simulink model "my_qpsk_simulink"  (R2022a)
settings: Solver=ode45  StartTime=0.0  StopTime=10.0  RelTol=1e-3  EnableMultiTasking=on
PreLoadFcn:
  | clc;
  | clear;
  | fs = 56e06;
  | f_clk = fs*6;
  | 
  | f_0 = 70e06;
  | f_c = f_0 - fs;
  | f_dds_out = f_c;
libraries: dsparch4 x4, dspxfrm3 x2, commchan3 x1, commsynccomp2 x1, commrandsrc2 x1, simulink x1, commdigbbndpm3 x1, dspsrcs4 x1
settings Model: Creator=laohe  LastModifiedBy=imlao
settings SolverCC: AlgebraicLoopSolver=TrustRegion
settings DataIOCC: LimitDataPoints=on  SaveFormat=Array  SignalLoggingSaveFormat=ModelDataLogs  ReturnWorkspaceOutputs=off
settings OptimizationCC: ExpressionDepthLimit=2147483647  LifeSpan=inf
settings DebuggingCC: UnderspecifiedInitializationDetection=Classic  MergeDetectMultiDrivingBlocksExec=none  SolverPrmCheckMsg=warning  FcnCallInpInsideContextMsg=warning  UnconnectedInputMsg=warning  UnconnectedOutputMsg=warning  UnconnectedLineMsg=warning  StateNameClashWarn=warning  SFUnexpectedBacktrackingDiag=warning  SFNoUnconditionalDefaultTransitionDiag=warning  SFExecutionAtInitializationDiag=none  SFMachineParentedDataDiag=warning  ArithmeticOperatorsInVariantConditions=warning
settings HardwareCC: ProdBitPerPointer=32  ProdBitPerSizeT=32  ProdBitPerPtrDiffT=32  ProdLargestAtomicFloat=None  ProdIntDivRoundTo=Undefined  ProdEndianess=Unspecified  ProdWordSize=32  ProdHWDeviceType=32-bit Generic
settings ModelReferenceCC: PropagateSignalLabelsOutOfModel=off
settings SFSimCC: SimUseLocalCustomCode=off  CustomCodeUndefinedFunction=UseInterfaceOnly
settings RTWCC: RTWUseLocalCustomCode=off
settings CodeAppCC: StateflowObjectComments=on
settings GRTTargetCC: TargetLangStandard=C89/C90 (ANSI)
settings ConfigComp: CovMetricSettings=dw  CovSaveCumulativeToWorkspaceVar=on  CovSaveSingleToWorkspaceVar=on  CovExternalEMLEnable=off

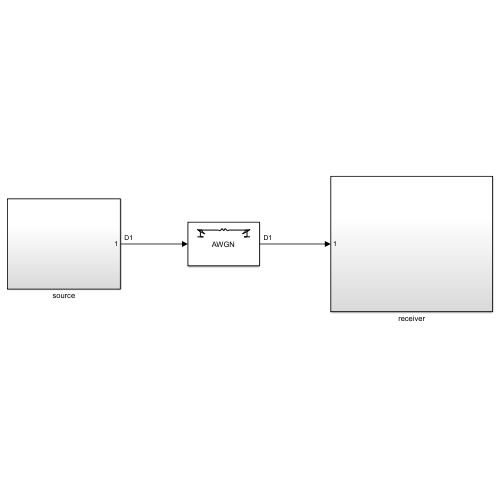
[thumbnail: Simulink's stored preview of the top-level diagram]
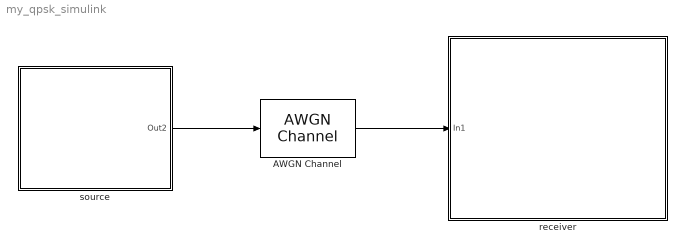
== system my_qpsk_simulink ==
  AWGN Channel : commchan3/AWGN Channel  InputProcessing=Columns as channels (frame based)  seed=67  noiseMode="Signal to noise ratio  (SNR)"  EbNodB=10  EsNodB=10  SNRdB=111  bitsPerSym=2  Ps=1  Tsym=1/2e06  variance=1
  receiver : Subsystem
  source : Subsystem
  wires:
  source/1(Out2) -> AWGN Channel/1
  AWGN Channel/1 -> receiver/1(In1)

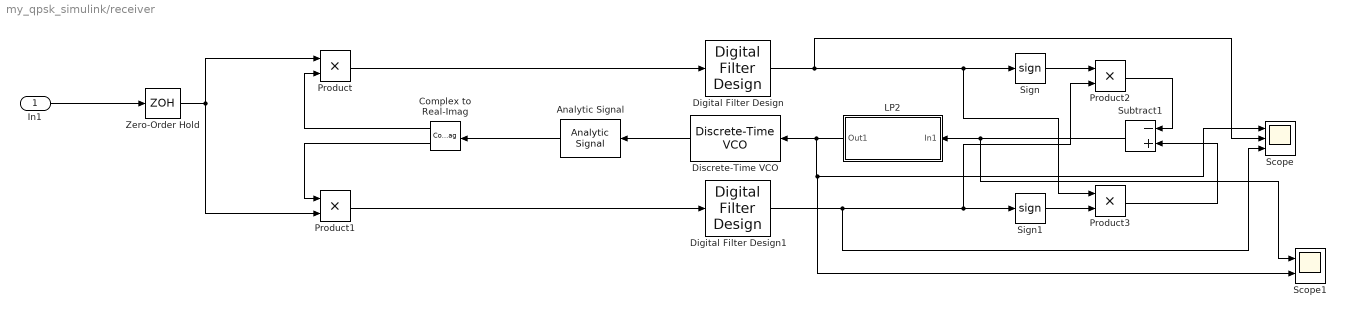
== system my_qpsk_simulink/receiver ==
  In1 : Inport
  Analytic Signal : dspxfrm3/Analytic Signal  N=100  InputProcessing=Columns as channels (frame based)
      settings: SourceProductBaseCode=DS
  Complex to Real-Imag : ComplexToRealImag
  Digital Filter Design : dsparch4/Digital Filter Design  mwdsp_browser_bugfix_var=off
  Digital Filter Design1 : dsparch4/Digital Filter Design  mwdsp_browser_bugfix_var=off
  Discrete-Time VCO : commsynccomp2/Discrete-Time VCO  Ac=1  Fc=f_dds_out  Kc=10000  Ph=0  ts=1/fs
      settings: SourceProductBaseCode=CM
  LP2 : Subsystem
  Product{,1..3} (4 alike) : Product  RndMeth=Zero
  Scope : Scope  NumInputPorts=3
  Scope1 : Scope  NumInputPorts=2
  Sign : Signum
  Sign1 : Signum
  Subtract1 : Sum  Inputs=-+
  Zero-Order Hold : ZeroOrderHold  SampleTime=1/fs
  wires:
  Analytic Signal/1 -> Complex to Real-Imag/1
  Complex to Real-Imag/1 -> Product/2
  Discrete-Time VCO/1 -> Analytic Signal/1
  Complex to Real-Imag/2 -> Product1/1
  In1/1 -> Zero-Order Hold/1
  Product1/1 -> Digital Filter Design1/1
  Product/1 -> Digital Filter Design/1
  Zero-Order Hold/1 -> Product1/2, Product/1
  Digital Filter Design/1 -> Scope/2, Product3/1, Sign/1
  LP2/1(Out1) -> Scope1/2, Scope/1, Discrete-Time VCO/1
  Sign/1 -> Product2/1
  Digital Filter Design1/1 -> Scope/3, Product2/2, Sign1/1
  Sign1/1 -> Product3/2
  Product2/1 -> Subtract1/1
  Product3/1 -> Subtract1/2
  Subtract1/1 -> Scope1/1, LP2/1(In1)

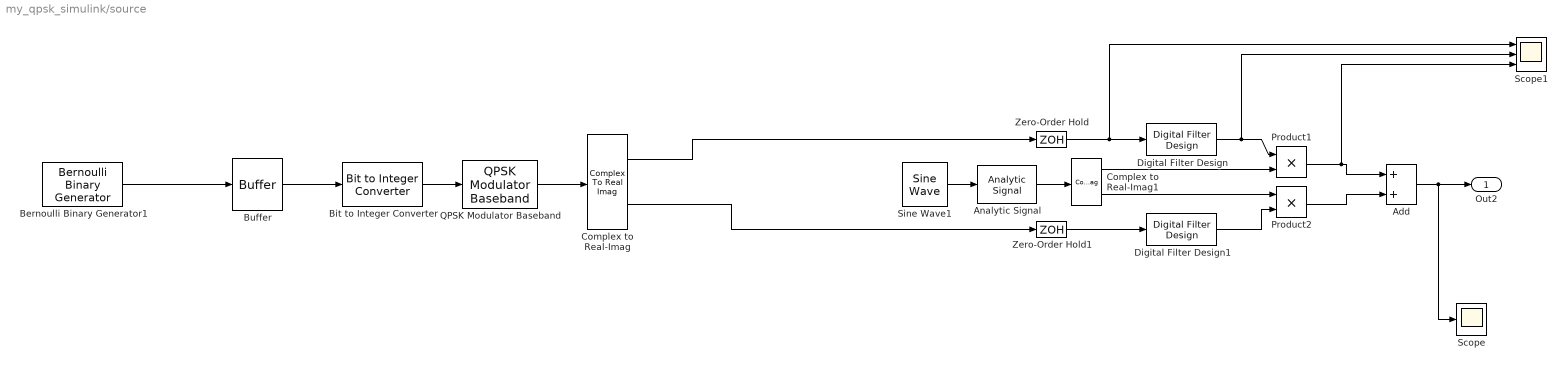
== system my_qpsk_simulink/source ==
  Add : Sum
  Analytic Signal : dspxfrm3/Analytic Signal  N=100  InputProcessing=Columns as channels (frame based)
      settings: SourceProductBaseCode=DS
  Bernoulli Binary Generator1 : commrandsrc2/Bernoulli Binary Generator  P=0.5  seed=61  Ts=1/2e06  frameBased=off  sampPerFrame=2  orient=off  outDataType=boolean
      settings: SourceProductBaseCode=CM
  Bit to Integer Converter : simulink/Logic and Bit Operations/Bit to Integer Converter  nbits=2  bitOrder=LSB first  signedOutputValues=Unsigned  outDtype=double  outDtypeSigned=Inherit via internal rule
      settings: SourceProductBaseCode=SL
  Buffer : Buffer  N=2  OutputFrames=off
  Complex to Real-Imag : ComplexToRealImag
  Complex to Real-Imag1 : ComplexToRealImag
  Digital Filter Design : dsparch4/Digital Filter Design  mwdsp_browser_bugfix_var=off
  Digital Filter Design1 : dsparch4/Digital Filter Design  mwdsp_browser_bugfix_var=off
  Product1 : Product  RndMeth=Zero
  Product2 : Product  RndMeth=Zero
  QPSK Modulator Baseband : commdigbbndpm3/QPSK Modulator Baseband  InType=Integer  Enc=Gray  Ph=0  outDtype=double  outWordLen=16  outUDDataType=sfix(16)  outFracLenMode=Best precision  outFracLen=15  outDataTypeStr=double  outLastDataTypeStr=double
  Scope : Scope
  Scope1 : Scope  NumInputPorts=3
  Sine Wave1 : dspsrcs4/Sine Wave  Amplitude=1  Frequency=f_c+1100  Phase=rand*2*pi  SampleMode=Discrete  OutComplex=Real  CompMethod=Trigonometric fcn  TableSize=Speed  SampleTime=1/fs  SamplesPerFrame=1  ResetState=Restart at time zero  OutputFrames=on  dataType=double  wordLen=16  udDataType=sfix(16)  fracBitsMode=Best precision  numFracBits=15  OutDataTypeStr=double  LastOutDataTypeStr=double
  Zero-Order Hold : ZeroOrderHold  SampleTime=1/fs
  Zero-Order Hold1 : ZeroOrderHold  SampleTime=1/fs
  Out2 : Outport
  wires:
  QPSK Modulator Baseband/1 -> Complex to Real-Imag/1
  Bernoulli Binary Generator1/1 -> Buffer/1
  Bit to Integer Converter/1 -> QPSK Modulator Baseband/1
  Sine Wave1/1 -> Analytic Signal/1
  Analytic Signal/1 -> Complex to Real-Imag1/1
  Complex to Real-Imag1/1 -> Product1/2
  Complex to Real-Imag1/2 -> Product2/1
  Product1/1 -> Scope1/3, Add/1
  Product2/1 -> Add/2
  Add/1 -> Scope/1, Out2/1
  Digital Filter Design/1 -> Scope1/2, Product1/1
  Zero-Order Hold/1 -> Scope1/1, Digital Filter Design/1
  Zero-Order Hold1/1 -> Digital Filter Design1/1
  Digital Filter Design1/1 -> Product2/2
  Complex to Real-Imag/2 -> Zero-Order Hold1/1
  Buffer/1 -> Bit to Integer Converter/1
  Complex to Real-Imag/1 -> Zero-Order Hold/1

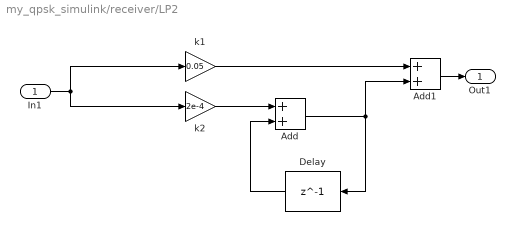
== system my_qpsk_simulink/receiver/LP2 ==
  In1 : Inport
  Add : Sum
  Add1 : Sum
  Delay : Delay  DelayLength=1  InitialCondition=0  InputProcessing=Columns as channels (frame based)
  k1 : Gain  Gain=0.05
  k2 : Gain  Gain=2e-4
  Out1 : Outport
  wires:
  k2/1 -> Add/1
  Add/1 -> Delay/1, Add1/2
  Delay/1 -> Add/2
  k1/1 -> Add1/1
  In1/1 -> k1/1, k2/1
  Add1/1 -> Out1/1
